simulink model "Lift_Q8"  (R2020a)
settings: Solver=VariableStepAuto  StartTime=0.0  StopTime=inf  RelTol=1e-3
settings Model: Creator=DELL  LastModifiedBy=DELL

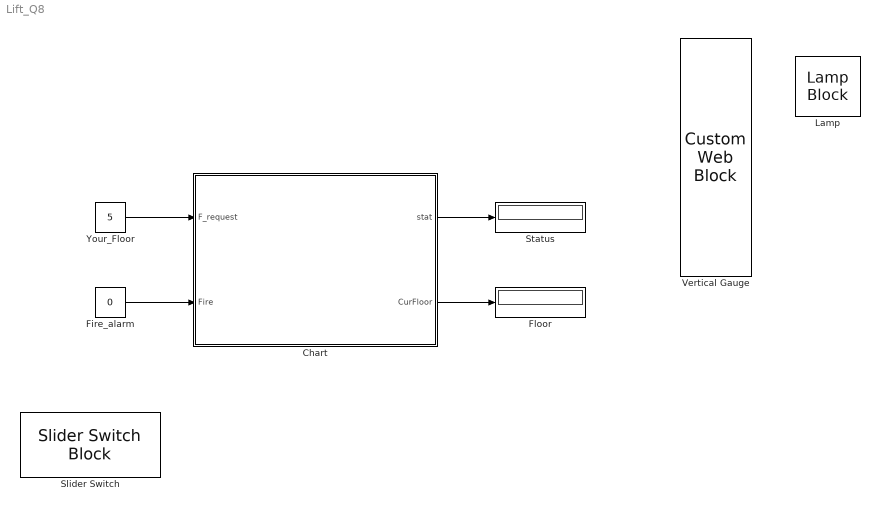
== system Lift_Q8 ==
  Chart : Stateflow chart  TreatAsAtomicUnit=on
  Fire_alarm : Constant  Value=0
  Floor : Display
  Lamp : LampBlock
  Slider Switch : SliderSwitchBlock
      settings: Values={{'Off', 'On'}, [0 1]}
  Status : Display
  Vertical Gauge : CustomWebBlock  ShowInitialText=on  Configuration="{\"components\":[{\"name\":\"LinearScaleComponent\",\"settings\":{\"bounds\":{\"max\":5,\"min\":0,\"tickInterval\":1},\"labelColor\":[250,245,199],\"labelFont\":{\"font\":\"Arial\",\"fontSize\":12},\"labelTransparency\":1,\"needleImage\":{\"size\":[21,75],\"src\":\"data:image\\/svg+xml;base64,PHN2ZyB4bWxucz0iaHR0cDovL3d3dy53My5vcmcvMjAwMC9zdmciIHhtbG5zOnhsaW5rPSJodHRwOi8vd3d3LnczLm9yZy8xOTk5L3hsaW5rIiB2aWV3Qm94PSIwIDAgMjEgNzUiPjxkZWZzPjxzdHlsZT4uY2xzLTF7ZmlsbDpub25lO30uY2xzLTJ7aXNvbGF0aW9uOmlzb2xhdGU7fS5jbHMtM3tjbGlwLXBhdGg6dXJsKCNjbGlwLXBhdGgpO30uY2xzLTR7b3BhY2l0eTowLjM7bWl4LWJsZW5kLW1vZGU6bXVsdGlwbHk7fS5jbHMtNXtmaWxsOiNlYjI2Mjk7fTwvc3R5bGU+PGNsaXBQYXRoIGlkPSJjbGlwLXBhdGgiIHRyYW5zZm9y ...(+1928 chars)\",\"srcOrientation\":\"horizontal\"},\"needleOffset\":[-0.01094391244870041,0],\"needleSize\":{\"height\":0.11960078534031414,\"width\":0.7589285714285714},\"position\":[0.015887605042016806,0.06986607142857143,0.8,0.9641544117647058],\"scaleColorSize\":0.24,\"scaleColors\":[],\"scaleColorsSize\":0.2,\"tickColor\":[250,245,200],\"tickTransparency\":1,\"valueBarColor\":[23,89,176],\"valueBarSize\":0.23,\"valueBarTransparency\":1}},{\"name\":\"BackgroundImageComponent\",\"settings\":{\"image\":{\"size\":[380,101],\"src\":\"data:image\\/svg+xml;base64,PHN2ZyB4bWxucz0iaHR0cDovL3d3dy53My5vcmcvMjAwMC9zdmciIHhtbG5zOnhsaW5rPSJodHRwOi8vd3d3LnczLm9yZy8xOTk5L3hsaW5rIiB2aWV3Qm94PSIwIDAgMzgwIDEwMSI+PGRlZnM+PHN0eWxlPi5jbHMtMXtmaWxsOnVybCgjbGluZWFyLWdyYWRpZW50KTt9LmNscy0ye2ZpbGw6dXJsKCNsaW5lYXItZ3JhZGllbnQtMik7fS5jbHMtM3tmaWxsOnVybCgjbGluZWFyLWdyYWRpZW50LTMpO308L3N0eWxlPjxsaW5lYXJHcmFkaWVudCBpZD0ibGluZWFyLWdyYWRpZW50IiB5MT0iNTAuNSIgeDI9IjM5OS4yOCIgeTI9IjUw ...(+2216 chars)\",\"srcOrientation\":\"horizontal\"},\"position\":[0,0,1,1],\"scaleMode\":\"0\"}}],\"settings\":{\"BindingType\":\"signal\",\"fixedAspectRatio\":\"on\",\"orientation\":\"vertical\"},\"type\":\"LinearGauge\"}"
  Your_Floor : Constant  Value=5
  wires:
  Chart/2(CurFloor) -> Floor/1
  Chart/1(stat) -> Status/1
  Your_Floor/1 -> Chart/1(F_request)
  Fire_alarm/1 -> Chart/2(Fire)

== stateflow chart Lift_Q8/Chart ==
  state Lift [parallel]
    entry:
    stat=0;
    settings: executionOrder=1
    state LiftOn
      (history)
      state GroundFloor
        entry:
        stat=1;
        during:
        CurFloor=0;
        FloorOperation(CurFloor);
        exit:
        stat=0;
      state FirstFloor
        entry:
        stat=1;
        during:
        CurFloor=1;
        FloorOperation(CurFloor);
        exit:
        stat=0;
      state SecondFloor
        entry:
        stat=1;
        during:
        CurFloor=2;
        FloorOperation(CurFloor);
        exit:
        stat=0;
      state ThirdFloor
        entry:
        stat=1;
        during:
        CurFloor=3;
        FloorOperation(CurFloor);
        exit:
        stat=0;
      state FourthFloor
        entry:
        stat=1;
        during:
        CurFloor=4;
        FloorOperation(CurFloor);
        exit:
        stat=0;
      state FifthFloor
        entry:
        stat=1;
        during:
        CurFloor=5;
        FloorOperation(CurFloor);
        exit:
        stat=0;
      (default) -> GroundFloor
      GroundFloor -> FirstFloor : FloorUp
      FirstFloor -> GroundFloor [order 2] : FloorDown
      FirstFloor -> SecondFloor [order 1] : FloorUp
      SecondFloor -> FirstFloor [order 2] : FloorDown
      SecondFloor -> ThirdFloor [order 1] : FloorUp
      ThirdFloor -> SecondFloor [order 2] : FloorDown
      ThirdFloor -> FourthFloor [order 1] : FloorUp
      FourthFloor -> ThirdFloor [order 2] : FloorDown
      FourthFloor -> FifthFloor [order 1] : FloorUp
      FifthFloor -> FourthFloor : FloorDown
    state LiftOff
      en:
      stat=0;
    (default) -> LiftOn
    LiftOff -> LiftOn : [Fire==0]
    LiftOn -> LiftOff : [Fire==1]
  state AlarmSet [parallel]
    settings: executionOrder=2
    (default) -> (junction 97) : {alarmStat=Fire;}
    (junction 97) -> (junction 100)
    (junction 100) -> (junction 102) [order 1] : [1]
    (junction 102) -> (junction 106) [order 2] : [alarmStat==1]{send(OpOff);}
    (junction 100) -> (junction 113) [order 2]
    (junction 102) -> (junction 104) [order 1] : [alarmStat==0]{send(OpOn);}
    (junction 106) -> (junction 108)
    (junction 108) -> (junction 104)
  state y = FloorOperation(floor) [function]
    (default) -> (junction 60)
    (junction 60) -> (junction 59) [order 3] : [F_request<floor]{
        | send(FloorDown);
        | disp('Down');}
    (junction 60) -> (junction 58) [order 1] : [F_request>floor]{
        | send(FloorUp);
        | disp('Up');}
    (junction 58) -> (junction 65)
    (junction 60) -> (junction 62) [order 2] : [F_request==floor]{
        | disp('CurrentFloor');}
    (junction 59) -> (junction 66)
    (junction 65) -> (junction 62)
    (junction 66) -> (junction 62)
    (junction 62) -> (junction 52)
  data: floor function_input; y function_output; stat output; CurFloor output; F_request input; Fire input; alarmStat local
  events: FloorUp local FUNCTION_CALL_EVENT; FloorDown local FUNCTION_CALL_EVENT; OpOn local FUNCTION_CALL_EVENT; OpOff local FUNCTION_CALL_EVENT
